simulink model "dual_quaternion_equation_of_motion_3"  (R2016a)
settings: Solver=VariableStepAuto  StartTime=0.0  StopTime=180  RelTol=1e-3
InitFcn:
  | addpath('..');
undefined symbols (not defined in the file or in its folder): F, MIL
libraries: aerolibconvert2 x16, aerolibwind2 x1, aerolibatmos2 x1, aerolibanim x1, simulink x1, aerolibtransform2 x1
settings Model: Creator=AkhramovichSA  LastModifiedBy=AkhramovichSA

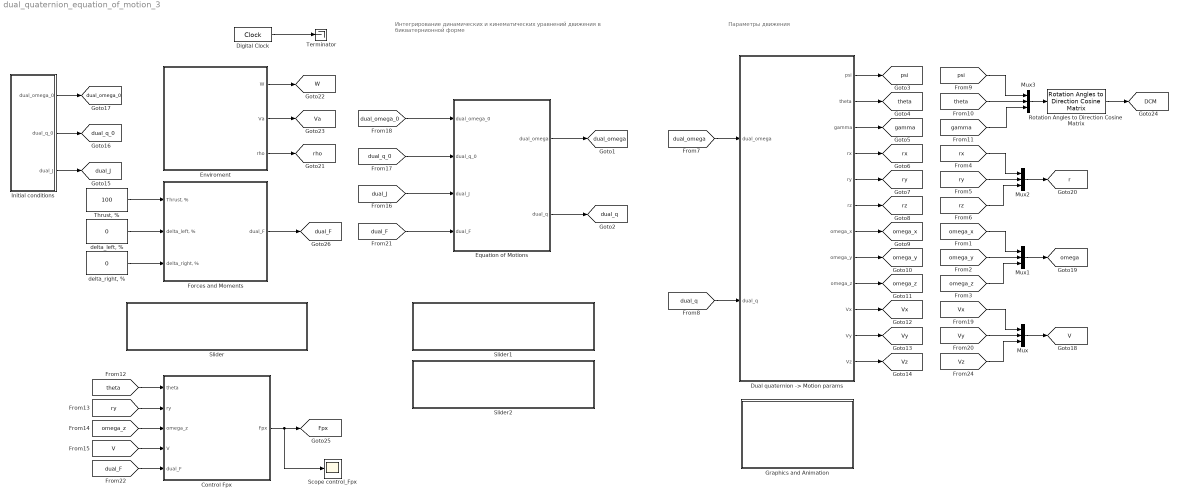
== system dual_quaternion_equation_of_motion_3 ==
  note: Интегрирование динамических и кинематических уравнений движения в бикватернионной форме
  note: Параметры движения
  Control Fpx : MATLAB Function  TreatAsAtomicUnit=on
  Digital Clock : DigitalClock
  "Dual quaternion -> Motion params" : MATLAB Function  TreatAsAtomicUnit=on
  Enviroment : Subsystem
  Equation of Motions : Subsystem
  Forces and Moments : Subsystem
  Graphics and Animation : Subsystem
  Initial conditions : Subsystem
  Mux{,1..3} (4 alike) : Mux  Inputs=3
  Rotation Angles to Direction Cosine Matrix : aerolibtransform2/Rotation Angles to Direction Cosine Matrix  rotationOrder=YZX
  Scope control_Fpx : Scope
  Slider : Subsystem  DialogController=hmiCreateDDGDialog  IsWebBlock=on  mask(MWDashboardBlock){webBlockId=836bae8a-61ff-49e9-8a0b-c22522f8dc87, webBlockType=slider, ShowInLibBrowser=on, ShowInitialText=on, HMISrcModelName=dual_quaternion_equation_of_motion_3}
      mask prompts: webBlockId "WebBlock Id"; webBlockType "WebBlock Type"; HMISrcModelName "Source Model"
      mask Help: helpview([docroot '/mapfiles/simulink.map'], 'hmi_slider')
      mask Display:
      | if strcmp(get_param(bdroot(gcb),'BlockDiagramType'), 'library')
      |     image([(matlabroot) '/toolbox/simulink/hmi/icons/Slider.png']);
      | end
  Slider1 : Subsystem  DialogController=hmiCreateDDGDialog  IsWebBlock=on  mask(MWDashboardBlock){webBlockId=4b1f0545-d665-4f13-8145-7b79bf56e625, webBlockType=slider, ShowInLibBrowser=on, ShowInitialText=on, HMISrcModelName=dual_quaternion_equation_of_motion_3}
      mask prompts: webBlockId "WebBlock Id"; webBlockType "WebBlock Type"; HMISrcModelName "Source Model"
      mask Help: helpview([docroot '/mapfiles/simulink.map'], 'hmi_slider')
      mask Display:
      | if strcmp(get_param(bdroot(gcb),'BlockDiagramType'), 'library')
      |     image([(matlabroot) '/toolbox/simulink/hmi/icons/Slider.png']);
      | end
  Slider2 : Subsystem  DialogController=hmiCreateDDGDialog  IsWebBlock=on  mask(MWDashboardBlock){webBlockId=93b55f6f-cf91-4fd5-b862-bc3a55f23f6b, webBlockType=slider, ShowInLibBrowser=on, ShowInitialText=on, HMISrcModelName=dual_quaternion_equation_of_motion_3}
      mask prompts: webBlockId "WebBlock Id"; webBlockType "WebBlock Type"; HMISrcModelName "Source Model"
      mask Help: helpview([docroot '/mapfiles/simulink.map'], 'hmi_slider')
      mask Display:
      | if strcmp(get_param(bdroot(gcb),'BlockDiagramType'), 'library')
      |     image([(matlabroot) '/toolbox/simulink/hmi/icons/Slider.png']);
      | end
  Terminator : Terminator
  "Thrust, %" : Constant  Value=100
  "delta_left, %" : Constant  Value=0
  "delta_right, %" : Constant  Value=0
  tag scope: DCM=global, Fpx=global, V=global, Va=global, Vx=global, Vy=global, Vz=global, W=global, dual_F=global, dual_J=global, dual_omega=global, dual_omega_0=global, dual_q=global, dual_q_0=global, gamma=global, omega=global, omega_x=global, omega_y=global, omega_z=global, psi=global, r=global, rho=global, rx=global, ry=global, rz=global, theta=global
  wires:
  Equation of Motions/1(dual_omega) -> [dual_omega]
  Equation of Motions/2(dual_q) -> [dual_q]
  [dual_omega] -> "Dual quaternion -> Motion params"/1(dual_omega)
  [dual_q] -> "Dual quaternion -> Motion params"/2(dual_q)
  "Dual quaternion -> Motion params"/1(psi) -> [psi]
  "Dual quaternion -> Motion params"/2(theta) -> [theta]
  "Dual quaternion -> Motion params"/3(gamma) -> [gamma]
  "Dual quaternion -> Motion params"/4(rx) -> [rx]
  "Dual quaternion -> Motion params"/5(ry) -> [ry]
  "Dual quaternion -> Motion params"/6(rz) -> [rz]
  "Dual quaternion -> Motion params"/7(omega_x) -> [omega_x]
  "Dual quaternion -> Motion params"/9(omega_z) -> [omega_z]
  "Dual quaternion -> Motion params"/8(omega_y) -> [omega_y]
  "Dual quaternion -> Motion params"/10(Vx) -> [Vx]
  "Dual quaternion -> Motion params"/11(Vy) -> [Vy]
  "Dual quaternion -> Motion params"/12(Vz) -> [Vz]
  "Thrust, %"/1 -> Forces and Moments/1("Thrust, %")
  [dual_J] -> Equation of Motions/3(dual_J)
  Initial conditions/3(dual_J) -> [dual_J]
  Initial conditions/2(dual_q_0) -> [dual_q_0]
  Initial conditions/1(dual_omega_0) -> [dual_omega_0]
  [dual_q_0] -> Equation of Motions/2(dual_q_0)
  [dual_omega_0] -> Equation of Motions/1(dual_omega_0)
  Digital Clock/1 -> Terminator/1
  "delta_left, %"/1 -> Forces and Moments/2("delta_left, %")
  "delta_right, %"/1 -> Forces and Moments/3("delta_right, %")
  [Vx] -> Mux/1
  [Vy] -> Mux/2
  [Vz] -> Mux/3
  Mux/1 -> [V]
  [omega_x] -> Mux1/1
  [omega_y] -> Mux1/2
  [omega_z] -> Mux1/3
  Mux1/1 -> [omega]
  [rx] -> Mux2/1
  [ry] -> Mux2/2
  [rz] -> Mux2/3
  Mux2/1 -> [r]
  Enviroment/1(W) -> [W]
  Enviroment/3(rho) -> [rho]
  Forces and Moments/1(dual_F) -> [dual_F]
  Enviroment/2(Va) -> [Va]
  Mux3/1 -> Rotation Angles to Direction Cosine Matrix/1
  [psi] -> Mux3/1
  [theta] -> Mux3/2
  [gamma] -> Mux3/3
  Rotation Angles to Direction Cosine Matrix/1 -> [DCM]
  [theta] -> Control Fpx/1(theta)
  [ry] -> Control Fpx/2(ry)
  [omega_z] -> Control Fpx/3(omega_z)
  [V] -> Control Fpx/4(V)
  Control Fpx/1(Fpx) -> Scope control_Fpx/1, [Fpx]
  [dual_F] -> Equation of Motions/4(dual_F)
  [dual_F] -> Control Fpx/5(dual_F)

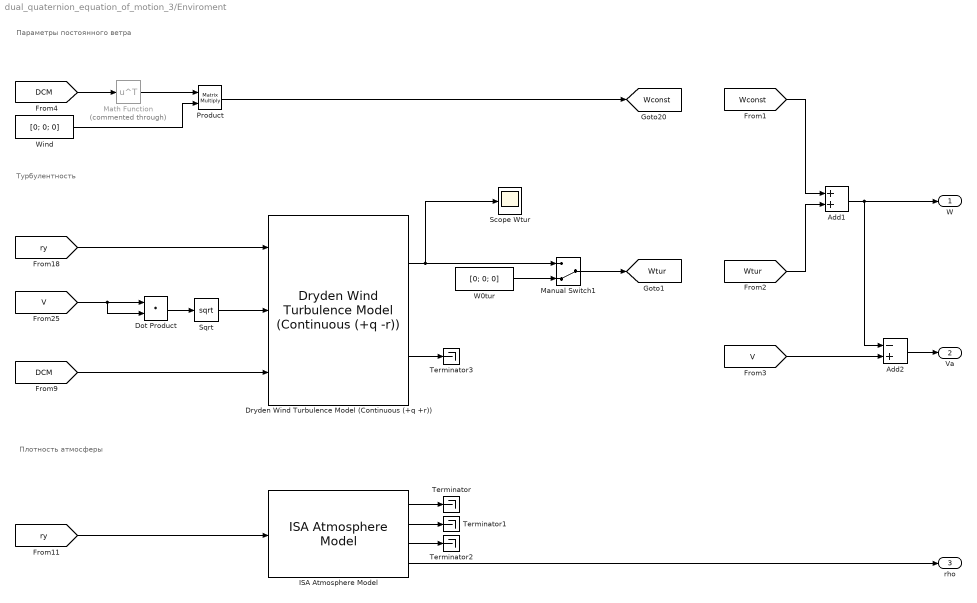
== system dual_quaternion_equation_of_motion_3/Enviroment ==
  note: Параметры постоянного ветра
  note: Турбулентность
  note: Плотность атмосферы
  Add1 : Sum
  Add2 : Sum  Inputs=-+
  Dot Product : DotProduct  InputSameDT=on  OutDataTypeStr=Inherit: Inherit via internal rule
  Dryden Wind Turbulence Model (Continuous (+q +r)) : aerolibwind2/Dryden Wind Turbulence Model  (Continuous (+q -r))  units=Metric (MKS)  spec=MIL-F-8785C  model=Continuous Dryden (+q +r)  W20=5  Wdeg=0  TurbProb=10^-1  L_high=533.4  Wingspan=10  ts=1  Seed=[23341 23342 23343 23344]  T_on=on
  ISA Atmosphere Model : aerolibatmos2/ISA Atmosphere Model  custom=off  g=9.80665  gamma=1.4  R=287.0531  L=0.0065  h_trop=11000  h_strat=20000  rho0=1.225  P0=101325  T0=288.15  h0=0
  Manual Switch1 : ManualSwitch  CurrentSetting=0
  Math Function : Math  Commented=through  Operator=transpose  SaturateOnIntegerOverflow=on
  Product : Product  Multiplication=Matrix(*)
  Scope Wtur : Scope
  Sqrt : Sqrt  SaturateOnIntegerOverflow=on
  Terminator{,1..3} (4 alike) : Terminator
  W0tur : Constant  Value=[0; 0; 0]
  Wind : Constant  Value=[0; 0; 0]
  W : Outport
  Va : Outport  Port=2
  rho : Outport  Port=3
  tag scope: Wconst=global, Wtur=global
  wires:
  [ry] -> ISA Atmosphere Model/1
  Dryden Wind Turbulence Model (Continuous (+q +r))/1 -> Scope Wtur/1, Manual Switch1/1
  [ry] -> Dryden Wind Turbulence Model (Continuous (+q +r))/1
  ISA Atmosphere Model/1 -> Terminator/1
  ISA Atmosphere Model/2 -> Terminator1/1
  ISA Atmosphere Model/3 -> Terminator2/1
  Dryden Wind Turbulence Model (Continuous (+q +r))/2 -> Terminator3/1
  W0tur/1 -> Manual Switch1/2
  Manual Switch1/1 -> [Wtur]
  [Wconst] -> Add1/1
  [Wtur] -> Add1/2
  Add1/1 -> Add2/1, W/1
  ISA Atmosphere Model/4 -> rho/1
  Add2/1 -> Va/1
  [V] -> Dot Product/2, Dot Product/1
  Dot Product/1 -> Sqrt/1
  Sqrt/1 -> Dryden Wind Turbulence Model (Continuous (+q +r))/2
  [V] -> Add2/2
  [DCM] -> Dryden Wind Turbulence Model (Continuous (+q +r))/3
  Product/1 -> [Wconst]
  Wind/1 -> Product/2
  [DCM] -> Math Function/1
  Math Function/1 -> Product/1

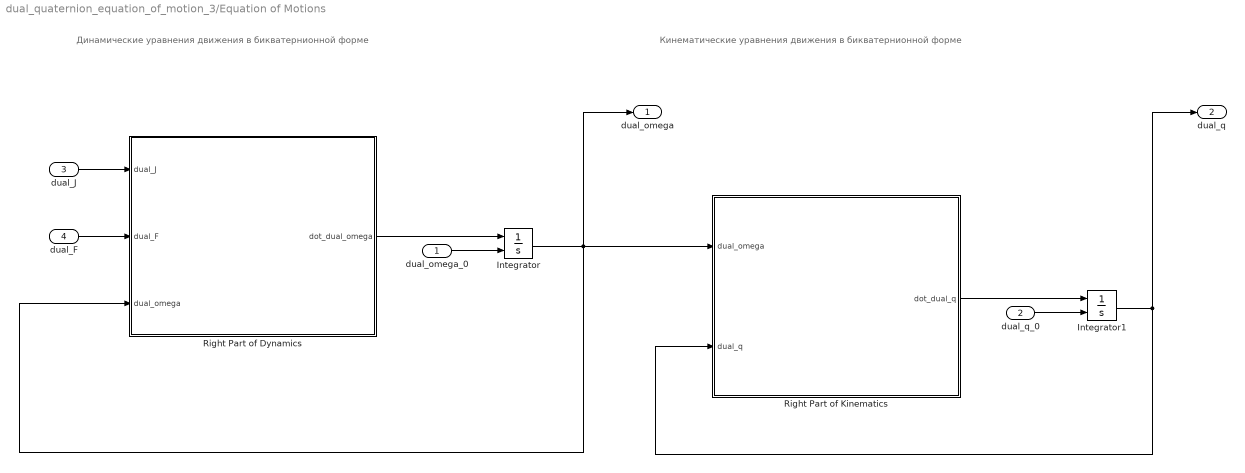
== system dual_quaternion_equation_of_motion_3/Equation of Motions ==
  note: Динамические уравнения движения в бикватернионной форме
  note: Кинематические уравнения движения в бикватернионной форме
  dual_omega_0 : Inport
  dual_q_0 : Inport  Port=2
  dual_J : Inport  Port=3
  dual_F : Inport  Port=4
  Integrator : Integrator  InitialConditionSource=external
  Integrator1 : Integrator  InitialConditionSource=external
  Right Part of Dynamics : MATLAB Function  TreatAsAtomicUnit=on
  Right Part of Kinematics : MATLAB Function  TreatAsAtomicUnit=on
  dual_omega : Outport
  dual_q : Outport  Port=2
  wires:
  Integrator/1 -> dual_omega/1, Right Part of Kinematics/1(dual_omega), Right Part of Dynamics/3(dual_omega)
  dual_omega_0/1 -> Integrator/2
  dual_q_0/1 -> Integrator1/2
  Right Part of Dynamics/1(dot_dual_omega) -> Integrator/1
  Integrator1/1 -> dual_q/1, Right Part of Kinematics/2(dual_q)
  dual_F/1 -> Right Part of Dynamics/2(dual_F)
  dual_J/1 -> Right Part of Dynamics/1(dual_J)
  Right Part of Kinematics/1(dot_dual_q) -> Integrator1/1

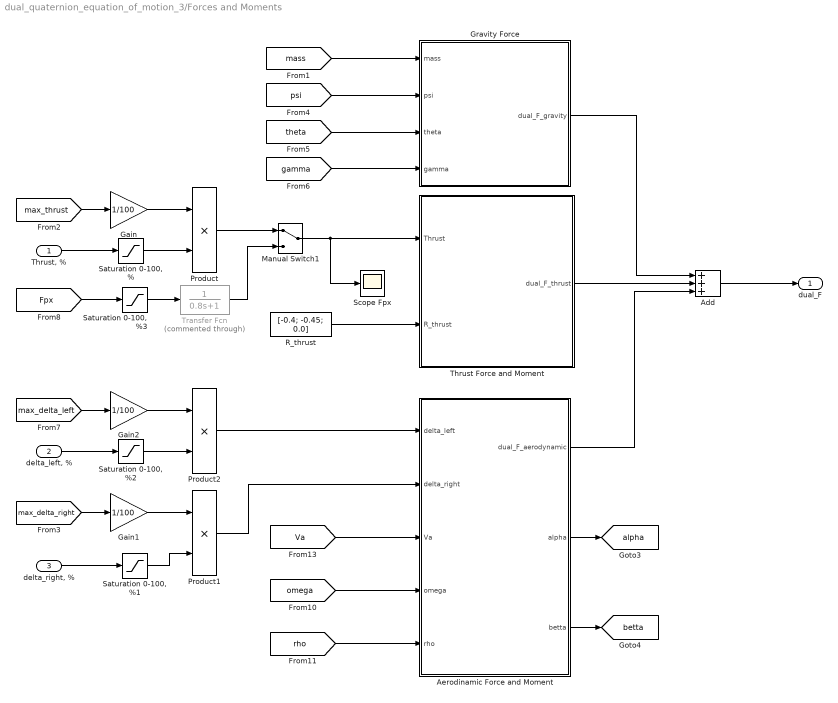
== system dual_quaternion_equation_of_motion_3/Forces and Moments ==
  "Thrust, %" : Inport
  "delta_left, %" : Inport  Port=2
  "delta_right, %" : Inport  Port=3
  Add : Sum  Inputs=+++
  Aerodinamic Force and Moment : MATLAB Function  TreatAsAtomicUnit=on
  Gain : Gain  Gain=1/100
  Gain1 : Gain  Gain=1/100
  Gain2 : Gain  Gain=1/100
  Gravity Force : MATLAB Function  TreatAsAtomicUnit=on
  Manual Switch1 : ManualSwitch
  Product : Product
  Product1 : Product
  Product2 : Product
  R_thrust : Constant  Value=[-0.4; -0.45; 0.0]
  "Saturation 0-100, %" : Saturate  UpperLimit=100  LowerLimit=0
  "Saturation 0-100, %1" : Saturate  UpperLimit=100  LowerLimit=0
  "Saturation 0-100, %2" : Saturate  UpperLimit=100  LowerLimit=0
  "Saturation 0-100, %3" : Saturate  UpperLimit=120  LowerLimit=0
  Scope Fpx : Scope
  Thrust Force and Moment : MATLAB Function  TreatAsAtomicUnit=on
  Transfer Fcn : TransferFcn  Commented=through  Denominator=[0.8 1]
  dual_F : Outport
  tag scope: alpha=global, betta=global
  wires:
  "Thrust, %"/1 -> "Saturation 0-100, %"/1
  [psi] -> Gravity Force/2(psi)
  [theta] -> Gravity Force/3(theta)
  [gamma] -> Gravity Force/4(gamma)
  [mass] -> Gravity Force/1(mass)
  R_thrust/1 -> Thrust Force and Moment/2(R_thrust)
  "Saturation 0-100, %"/1 -> Product/2
  [max_thrust] -> Gain/1
  Gain/1 -> Product/1
  [Va] -> Aerodinamic Force and Moment/3(Va)
  Aerodinamic Force and Moment/2(alpha) -> [alpha]
  Aerodinamic Force and Moment/3(betta) -> [betta]
  Gravity Force/1(dual_F_gravity) -> Add/1
  Add/1 -> dual_F/1
  "delta_right, %"/1 -> "Saturation 0-100, %1"/1
  "Saturation 0-100, %1"/1 -> Product1/2
  Product1/1 -> Aerodinamic Force and Moment/2(delta_right)
  [max_delta_right] -> Gain1/1
  Gain1/1 -> Product1/1
  "delta_left, %"/1 -> "Saturation 0-100, %2"/1
  "Saturation 0-100, %2"/1 -> Product2/2
  [max_delta_left] -> Gain2/1
  Gain2/1 -> Product2/1
  Product2/1 -> Aerodinamic Force and Moment/1(delta_left)
  [omega] -> Aerodinamic Force and Moment/4(omega)
  Thrust Force and Moment/1(dual_F_thrust) -> Add/2
  Aerodinamic Force and Moment/1(dual_F_aerodynamic) -> Add/3
  [rho] -> Aerodinamic Force and Moment/5(rho)
  "Saturation 0-100, %3"/1 -> Transfer Fcn/1
  [Fpx] -> "Saturation 0-100, %3"/1
  Product/1 -> Manual Switch1/1
  Transfer Fcn/1 -> Manual Switch1/2
  Manual Switch1/1 -> Scope Fpx/1, Thrust Force and Moment/1(Thrust)

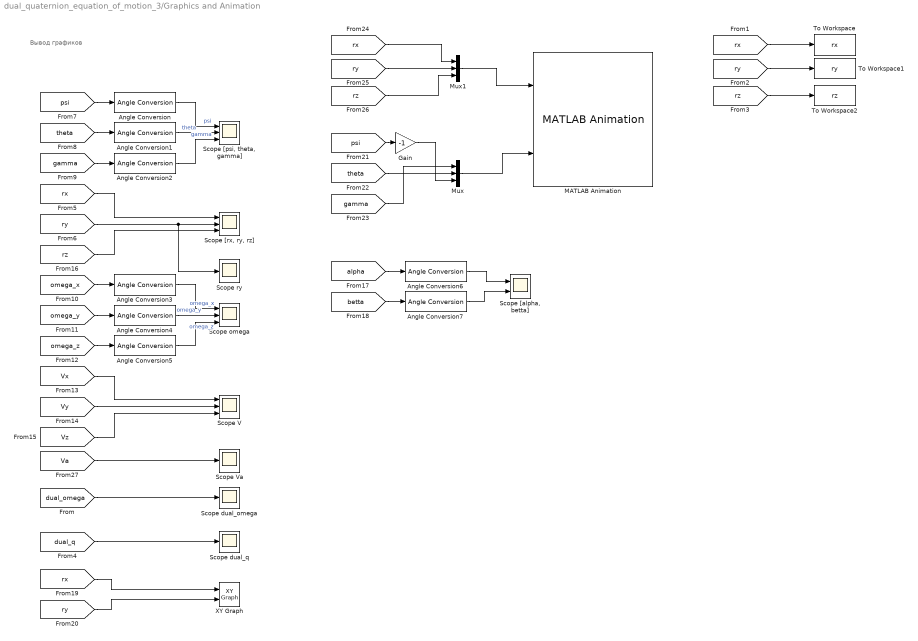
== system dual_quaternion_equation_of_motion_3/Graphics and Animation ==
  note: Вывод графиков
  Angle Conversion{,1..7} (8 alike) : aerolibconvert2/Angle Conversion  IU=rad  OU=deg
  Gain : Gain  Gain=-1
  MATLAB Animation : aerolibanim/MATLAB Animation  Tag=Matlab Animation 6 DOF  Vehicles=1  Geometries='astredwedge.mat'  BoundingBoxCoordinates=[-500,500,-500,500,-500,500]  CameraOffset=[0,100,0]  CameraViewAngle=10  SampleTime=0.2  FigurePosition=[552,86,532,373]
  Mux : Mux  Inputs=3
  Mux1 : Mux  Inputs=3
  Scope V : Scope  NumInputPorts=3
  Scope Va : Scope
  "Scope [alpha, betta]" : Scope  NumInputPorts=2
  "Scope [psi, theta, gamma]" : Scope  NumInputPorts=3
  "Scope [rx, ry, rz]" : Scope  NumInputPorts=3
  Scope dual_omega : Scope
  Scope dual_q : Scope
  Scope omega : Scope  NumInputPorts=3
  Scope ry : Scope
  To Workspace : ToWorkspace  VariableName=rx  SampleTime=-1
  To Workspace1 : ToWorkspace  VariableName=ry  SampleTime=-1
  To Workspace2 : ToWorkspace  VariableName=rz  SampleTime=-1
  XY Graph : simulink/Sinks/XY Graph  xmin=-1  xmax=1500  ymin=-1  ymax=120  st=-1
  wires:
  [ry] -> Mux1/2
  Mux/1 -> MATLAB Animation/2
  Mux1/1 -> MATLAB Animation/1
  [theta] -> Mux/2
  [rx] -> Mux1/1
  [rz] -> Mux1/3
  [ry] -> To Workspace1/1
  [rx] -> To Workspace/1
  [rz] -> To Workspace2/1
  [dual_omega] -> Scope dual_omega/1
  [dual_q] -> Scope dual_q/1
  [rx] -> "Scope [rx, ry, rz]"/1
  [ry] -> Scope ry/1, "Scope [rx, ry, rz]"/2
  [rz] -> "Scope [rx, ry, rz]"/3
  [Vx] -> Scope V/1
  [Vy] -> Scope V/2
  [Vz] -> Scope V/3
  [rx] -> XY Graph/1
  [ry] -> XY Graph/2
  [psi] -> Angle Conversion/1
  [theta] -> Angle Conversion1/1
  [gamma] -> Angle Conversion2/1
  Angle Conversion/1 -> "Scope [psi, theta, gamma]"/1  "psi"
  Angle Conversion1/1 -> "Scope [psi, theta, gamma]"/2  "theta"
  Angle Conversion2/1 -> "Scope [psi, theta, gamma]"/3  "gamma"
  Angle Conversion3/1 -> Scope omega/1  "omega_x"
  Angle Conversion4/1 -> Scope omega/2  "omega_y"
  Angle Conversion5/1 -> Scope omega/3  "omega_z"
  [omega_x] -> Angle Conversion3/1
  [omega_y] -> Angle Conversion4/1
  [omega_z] -> Angle Conversion5/1
  [alpha] -> Angle Conversion6/1
  [betta] -> Angle Conversion7/1
  Angle Conversion6/1 -> "Scope [alpha, betta]"/1
  Angle Conversion7/1 -> "Scope [alpha, betta]"/2
  [gamma] -> Mux/1
  Gain/1 -> Mux/3
  [psi] -> Gain/1
  [Va] -> Scope Va/1

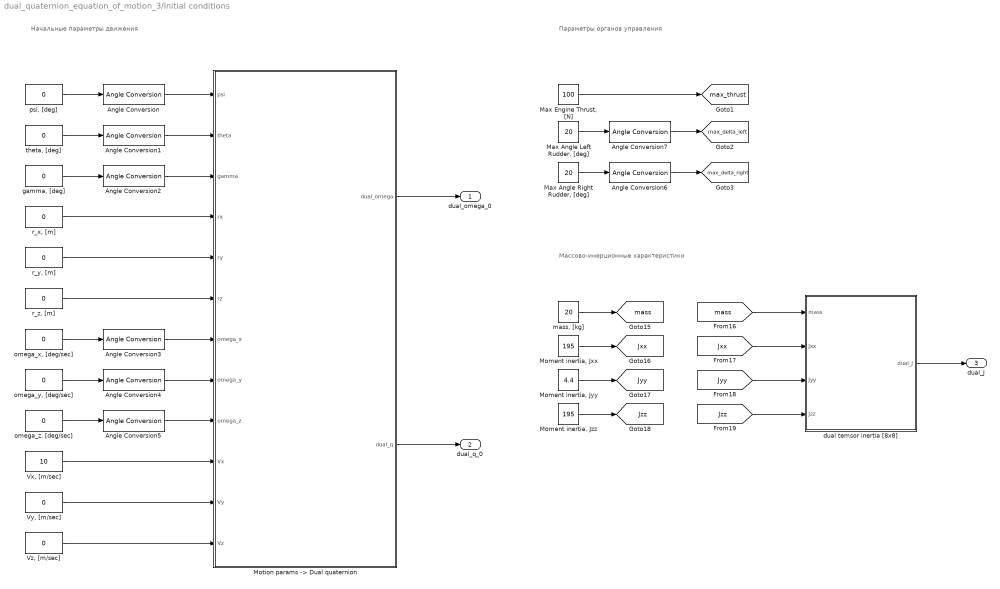
== system dual_quaternion_equation_of_motion_3/Initial conditions ==
  note: Начальные параметры движения
  note: Параметры органов управления
  note: Массово-инерционные характеристики
  Angle Conversion{,1..7} (8 alike) : aerolibconvert2/Angle Conversion  IU=deg  OU=rad
  "Max Angle Left Rudder, [deg]" : Constant  Value=20
  "Max Angle Right Rudder, [deg]" : Constant  Value=20
  "Max Engine Thrust, [N]" : Constant  Value=100
  "Moment inertia, Jxx" : Constant  Value=195
  "Moment inertia, Jyy" : Constant  Value=4.4
  "Moment inertia, Jzz" : Constant  Value=195
  "Motion params -> Dual quaternion" : MATLAB Function  TreatAsAtomicUnit=on
  "Vx, [m/sec]" : Constant  Value=10  VectorParams1D=off
  "Vy, [m/sec]" : Constant  Value=0  VectorParams1D=off
  "Vz, [m/sec]" : Constant  Value=0  VectorParams1D=off
  dual temsor inertia [8x8] : MATLAB Function  TreatAsAtomicUnit=on
  "gamma, [deg]" : Constant  Value=0  VectorParams1D=off
  "mass, [kg]" : Constant  Value=20
  "omega_x, [deg/sec]" : Constant  Value=0  VectorParams1D=off
  "omega_y, [deg/sec]" : Constant  Value=0  VectorParams1D=off
  "omega_z, [deg/sec]" : Constant  Value=0  VectorParams1D=off
  "psi, [deg]" : Constant  Value=0  VectorParams1D=off
  "r_x, [m]" : Constant  Value=0  VectorParams1D=off
  "r_y, [m]" : Constant  Value=0  VectorParams1D=off
  "r_z, [m]" : Constant  Value=0  VectorParams1D=off
  "theta, [deg]" : Constant  Value=0  VectorParams1D=off
  dual_omega_0 : Outport
  dual_q_0 : Outport  Port=2
  dual_J : Outport  Port=3
  tag scope: Jxx=global, Jyy=global, Jzz=global, mass=global, max_delta_left=global, max_delta_right=global, max_thrust=global
  wires:
  "psi, [deg]"/1 -> Angle Conversion/1
  "theta, [deg]"/1 -> Angle Conversion1/1
  "gamma, [deg]"/1 -> Angle Conversion2/1
  "r_x, [m]"/1 -> "Motion params -> Dual quaternion"/4(rx)
  "r_y, [m]"/1 -> "Motion params -> Dual quaternion"/5(ry)
  "r_z, [m]"/1 -> "Motion params -> Dual quaternion"/6(rz)
  "Motion params -> Dual quaternion"/1(dual_omega) -> dual_omega_0/1
  "Motion params -> Dual quaternion"/2(dual_q) -> dual_q_0/1
  "omega_x, [deg/sec]"/1 -> Angle Conversion3/1
  "omega_y, [deg/sec]"/1 -> Angle Conversion4/1
  "omega_z, [deg/sec]"/1 -> Angle Conversion5/1
  "Vx, [m/sec]"/1 -> "Motion params -> Dual quaternion"/10(Vx)
  "Vy, [m/sec]"/1 -> "Motion params -> Dual quaternion"/11(Vy)
  "Vz, [m/sec]"/1 -> "Motion params -> Dual quaternion"/12(Vz)
  Angle Conversion/1 -> "Motion params -> Dual quaternion"/1(psi)
  Angle Conversion1/1 -> "Motion params -> Dual quaternion"/2(theta)
  Angle Conversion2/1 -> "Motion params -> Dual quaternion"/3(gamma)
  Angle Conversion3/1 -> "Motion params -> Dual quaternion"/7(omega_x)
  Angle Conversion4/1 -> "Motion params -> Dual quaternion"/8(omega_y)
  Angle Conversion5/1 -> "Motion params -> Dual quaternion"/9(omega_z)
  "mass, [kg]"/1 -> [mass]
  "Moment inertia, Jxx"/1 -> [Jxx]
  "Moment inertia, Jyy"/1 -> [Jyy]
  "Moment inertia, Jzz"/1 -> [Jzz]
  [mass] -> dual temsor inertia [8x8]/1(mass)
  [Jxx] -> dual temsor inertia [8x8]/2(Jxx)
  [Jyy] -> dual temsor inertia [8x8]/3(Jyy)
  [Jzz] -> dual temsor inertia [8x8]/4(Jzz)
  dual temsor inertia [8x8]/1(dual_J) -> dual_J/1
  "Max Engine Thrust, [N]"/1 -> [max_thrust]
  "Max Angle Right Rudder, [deg]"/1 -> Angle Conversion6/1
  Angle Conversion6/1 -> [max_delta_right]
  "Max Angle Left Rudder, [deg]"/1 -> Angle Conversion7/1
  Angle Conversion7/1 -> [max_delta_left]

== system dual_quaternion_equation_of_motion_3/Slider ==

== system dual_quaternion_equation_of_motion_3/Slider1 ==

== system dual_quaternion_equation_of_motion_3/Slider2 ==

== matlab function dual_quaternion_equation_of_motion_3/Initial conditions/Motion params -> Dual quaternion ==
  data: psi input; dual_omega output; dual_q output; theta input; gamma input; rx input; ry input; rz input; omega_x input; omega_y input; omega_z input; Vx input; Vy input; Vz input
function [dual_omega, dual_q] = motion_params_to_dual_quaternion(psi, theta, gamma, rx, ry, rz, omega_x, omega_y, omega_z, Vx, Vy, Vz)
% Перевод параметров движения в бикватернионную форму

coder.extrinsic('dq_from_euler_translation'); % for simulink

dual_q     = [1; zeros(7, 1)];

dual_omega = [0; omega_x; omega_y; omega_z;  0; Vx; Vy; Vz];  % Начальная углоавя и линейная скорости
dual_q     = dq_from_euler_translation([psi; theta; gamma], [rx; ry; rz]);      % Начальное ориентация и положение ЛА

== matlab function dual_quaternion_equation_of_motion_3/Equation of Motions/Right Part of Dynamics ==
  data: dual_J input; dual_F input; dual_omega input; dot_dual_omega output
function dot_dual_omega  = dot_dual_omega(dual_J, dual_F, dual_omega)
% Правые части динамического уравнения движения в бикватернионной форме
% Выходные данные надо проинтегрировать звеном: 1/s

% Входные данные:
%
% Бикватернион угловых и линейных скоростей
% dual_omega = [0; omega_x; omega_y; omega_z; 0; v_x; v_y; v_z]
% 
% Бикватернион моментов и сил
% dual_F     = [0; Mx; My; Mz; 0; Fx; Fy; Fz]
%
% Расширенный тензор инерции в бикватернионной форме
% dual_J     = [1  0   0   0  0  0  0  0;
%               0 Jxx Jxy Jxz 0  0  0  0;
%               0 Jyx Jyy Jyz 0  0  0  0;
%               0 Jzx Jzy Jzz 0  0  0  0;
%               0  0   0   0  1  0  0  0;
%               0  0   0   0  0  m  0  0;
%               0  0   0   0  0  0  m  0;
%               0  0   0   0  0  0  0  m]
% 
% Выходные данные:
% 
% Правая часть дифференциального уравнения динамики, изменение бикватерниона угловых и линейных скоростей
% dot_dual_omega = [0; omega_x; omega_y; omega_z; 0; v_x; v_y; v_z]

dot_dual_omega = dual_J \ (dual_F - dq_cross([dual_omega(1:4); 0; 0; 0; 0], (dual_J*dual_omega)));

== matlab function dual_quaternion_equation_of_motion_3/Forces and Moments/Gravity Force ==
  data: mass input; dual_F_gravity output; psi input; theta input; gamma input
function dual_F_gravity = force_gravity(mass, psi, theta, gamma)

F_gravity_nsk = [0; -9.807*mass; 0];

F_gravity     = nsk2ssk(gamma, psi, theta)*F_gravity_nsk;

dual_F_gravity = [0; 0; 0; 0; 0; F_gravity];

== matlab function dual_quaternion_equation_of_motion_3/Forces and Moments/Thrust Force and Moment ==
  data: Thrust input; dual_F_thrust output; R_thrust input
function dual_F_thrust = Thrust_M_F(Thrust, R_thrust)

F_thrust = [Thrust; 0; 0];           % Сила и направление силы в ССК

% R_thrust = [-0.1; -0.2; 0.0];      % Точка приложения силы в ССК

M_thrust = cross(R_thrust, F_thrust);       % Момент в ССК
M_thrust = M_thrust + 0*[0; -Thrust*0.0; 0]; % Момент от винта

dual_F_thrust = [0; M_thrust; 0; F_thrust];

% 100 %  -//- 10 N (max)
%  70 %  -//- x 
% x = 10*70/100

== matlab function dual_quaternion_equation_of_motion_3/Dual quaternion -> Motion params ==
  data: dual_omega input; psi output; theta output; dual_q input; gamma output; rx output; ry output; rz output; omega_x output; omega_y output; omega_z output; Vx output; Vy output; Vz output
function [psi, theta, gamma, rx, ry, rz, omega_x, omega_y, omega_z, Vx, Vy, Vz] = dual_quaternion_to_motion_params(dual_omega, dual_q)
% Перевод в бикватернионна скорости и положения в параметры движения

coder.extrinsic('dq_get_rotation_euler', 'dq_get_translation_vector'); % for simulink

omega   = dual_omega(2:4); % Угловая скорость, [рад/с]
omega_x = omega(1);
omega_y = omega(2);
omega_z = omega(3);

V  = dual_omega(6:8); % Линейная скорость, [м/с]
Vx = V(1);
Vy = V(2);
Vz = V(3);

psi   = 0;
theta = 0;
gamma = 0;
[psi, theta, gamma] = dq_get_rotation_euler(dual_q);     % Углы ориентации, [рад]

r  = zeros(3,1);
r  = dq_get_translation_vector(dual_q); % Радиус-вектор положения ЛА, [м]
rx = r(1);
ry = r(2);
rz = r(3);

== matlab function dual_quaternion_equation_of_motion_3/Initial conditions/dual temsor inertia [8x8] ==
  data: mass input; dual_J output; Jxx input; Jyy input; Jzz input
function dual_J = dual_J(mass, Jxx, Jyy, Jzz)

dual_J = [1  0  0  0  0  0   0   0; 
          0 Jxx 0  0  0  0   0   0; 
          0  0 Jyy 0  0  0   0   0; 
          0  0  0 Jzz 0  0   0   0; 
          0  0  0  0  1  0   0   0; 
          0  0  0  0  0 mass 0   0; 
          0  0  0  0  0  0  mass 0; 
          0  0  0  0  0  0   0  mass];

== matlab function dual_quaternion_equation_of_motion_3/Forces and Moments/Aerodinamic Force and Moment ==
  data: delta_left input; dual_F_aerodynamic output; delta_right input; Va input; omega input; alpha output; betta output; rho input
function [dual_F_aerodynamic, alpha, betta] = Aerodinamic_M_F(delta_left, delta_right, Va, omega, rho)

S  = 10.5;  % Площадь крыла, м^2
ba = 1;     % Средняя аэродинамичекая хорда (САХ)
% rho = 1.225;

omega_x = omega(1);
omega_y = omega(2);
omega_z = omega(3);

% W       = nsk2ssk(gamma, psi, theta)'*W;
% W       = W + Wtur;

% Va      = V - W;                             % Вектор воздушнной скорости, [м/с]
Va_norm = sqrt(Va(1)^2 + Va(2)^2 + Va(3)^2); % Воздушная скорость, [м/с]
q       = (rho*Va_norm^2)/2;                 % Скоростной напор, [кг/(м*с^2)]
alpha   = atan(-Va(2)/Va(1)) + deg2rad(0);   % Угол атаки, [рад]
betta   = asin(Va(3)/Va_norm);               % Угол скольжения, [рад]

% Управление стропами, рули отклоняются только вниз в полжительном направлении от 0 до 20 градусов.
% delta_left  = deg2rad(0.0); % Угол отклонения левого руля, [рад]
% delta_right = deg2rad(0.0); % Угол отклонения правого руля, [рад]

% Управляющие воздействия вокруг по каждой из осей, [рад]
delta_x = 0.5*(delta_left  - delta_right);
delta_y = 0.5*(delta_right - delta_left);
delta_z = 0.5*(delta_left  + delta_right);

% Аэродинамические коэфициенты
% Коеффициенты силы сопротивления
cx_alpha_0 = 0.08 + 0.1;
cx_alpha   = 0.05;
cx_alpha_2 = 1.1;
cx_delta   = 0.0;

% Коеффициенты подъемной силы
cy_alpha_0 = 0.15;
cy_alpha   = 3.8;
cy_delta   = 0.8;

% Коеффициенты боковой силы
cz_betta_0 =  0.0;
cz_betta   = -0.11;
cz_delta   =  0.0;

% Коеффициенты момента крена
mx_betta_0 =  0.0;
mx_betta   = -0.5;
mx_alpha   =  0.0;
mx_delta   =  0.0;
mx_omega_x = -1.5;
mx_omega_y = -1.0;
mx_omega_z =  0.0;

% Коеффициенты момента рысканья
my_betta_0 =  0.0;
my_betta   =  -0.8;
my_delta   =  -1.5;
my_omega_y_0     = -10.0;
my_omega_y_betta = -10.0;

% Коеффициенты момента тангажа
mz_alpha_0 = 0.3; % -0.08;
mz_alpha   = -3.0;
% mz_alpha_2 = -10.0;
mz_delta   =  -0.4;
mz_omega_z_0     = -4.0;
mz_omega_z_alpha = -0.5;


%% 
cx = cx_alpha_0 + cx_alpha*alpha + cx_alpha_2*alpha^2;
cy = cy_alpha_0 + cy_alpha*alpha + cy_delta*delta_z;
cz = cz_betta_0 + cz_betta*betta + cz_delta*delta_y;

% mx = mx_betta_0 + mx_betta*betta + mx_delta*delta_x;
% my = my_betta_0 + my_betta*betta + my_delta*delta_y;
% mz = mz_alpha_0 + mz_alpha*alpha + mz_delta*delta_z; % + mz_alpha_2*alpha^2 ;

mx = mx_betta_0 + mx_betta*betta + mx_alpha*alpha + mx_omega_x*(ba/Va_norm)*omega_x + mx_omega_y*(ba/Va_norm)*omega_y + mx_omega_z*(ba/Va_norm)*omega_z + mx_delta*delta_x;
my = my_betta_0 + my_betta*betta + (my_omega_y_0 + my_omega_y_betta*betta)*(ba/Va_norm)*omega_y + my_delta*delta_y;
mz = mz_alpha_0 + mz_alpha*alpha + (mz_omega_z_0 + mz_omega_z_alpha*alpha)*(ba/Va_norm)*omega_z + mz_delta*delta_z;

Fa_pssk = [-cx; cy; cz]*q*S;          % вектор аэродинамической силы в ПССК

Fa = pssk2ssk(alpha, betta)*Fa_pssk;  % перевод в ССК
Ma = [mx; my; mz]*q*ba*S;             % момент в ПССК

dual_F_aerodynamic = [0; Ma; 0; Fa];

== matlab function dual_quaternion_equation_of_motion_3/Equation of Motions/Right Part of Kinematics ==
  data: dual_omega input; dual_q input; dot_dual_q output
function dot_dual_q  = dot_dual_q(dual_omega, dual_q)
% Правые части кинематического уравнения движения в бикватернионной форме
% Выходные данные надо проинтегрировать звеном: 1/s

% Входные данные:
%
% Бикватернион угловых и линейных скоростей
% dual_omega = [0; omega_x; omega_y; omega_z; 0; v_x; v_y; v_z]
%
% Бикватернион углового и линейного положения
% dual_q     = [q1; q2; q3; q4; q5; q6; q7; q8]
% 
% Выходные данные:
% 
% Правая часть дифференциального уравнения кинематики, изменение бикватерниона углового и линейного положения
% dot_dual_q     = [q1; q2; q3; q4; q5; q6; q7; q8]

dot_dual_q     = 0.5*dq_multiply(dual_q, dual_omega);

== matlab function dual_quaternion_equation_of_motion_3/Control Fpx ==
  data: theta input; ry input; Fpx output; omega_z input; V input; dual_F input
function Fpx = control_Fpx(theta, ry, omega_z, V, dual_F)

Vx = V(1);
Vy = V(2);

Jzz = 195;
ly = -0.45;

Maz = dual_F(4);

k1 = 10.0;
k2 = 5.0;
k3 = 0.01;

Fpx = (Jzz/ly)*(Maz/Jzz + (ry - 110)*((k1*k2*k3)/Vx + k1/Vx +k3*Vx) + ... 
             (theta + Vy/Vx)*(1 + Vx^2 + k1*k2 + k2*k3 + k1*k3) + ...
             omega_z*(k1 + k2 + k3));
